simulink model "TST_LogicOperations"  (Simulink 10.0)
settings: Solver=FixedStepDiscrete  StartTime=0.0  StopTime=10.0  FixedStep=0.02  RelTol=1e-3  EnableMultiTasking=on
settings Model: Creator=kharthforeign  LastModifiedBy=unknown
settings DataIOCC: LimitDataPoints=on  SignalLoggingSaveFormat=ModelDataLogs  SaveOutput=off  SignalLogging=off  SaveTime=off
settings OptimizationCC: BlockReduction=off  ConditionallyExecuteInputs=off  OptimizeBlockIOStorage=off  BufferReuse=off  GlobalBufferReuse=off  ExpressionFolding=off  ExpressionDepthLimit=2147483647  LocalBlockOutputs=off  InitFltsAndDblsToZero=on  OptimizeDataStoreBuffers=off  BusAssignmentInplaceUpdate=off
settings DebuggingCC: SolverPrmCheckMsg=warning  FcnCallInpInsideContextMsg=warning  StateNameClashWarn=warning
settings SFSimCC: SimParseCustomCode=off
settings GRTTargetCC: GeneratePreprocessorConditionals=Disable all
settings ConfigComp: CovExternalEMLEnable=off

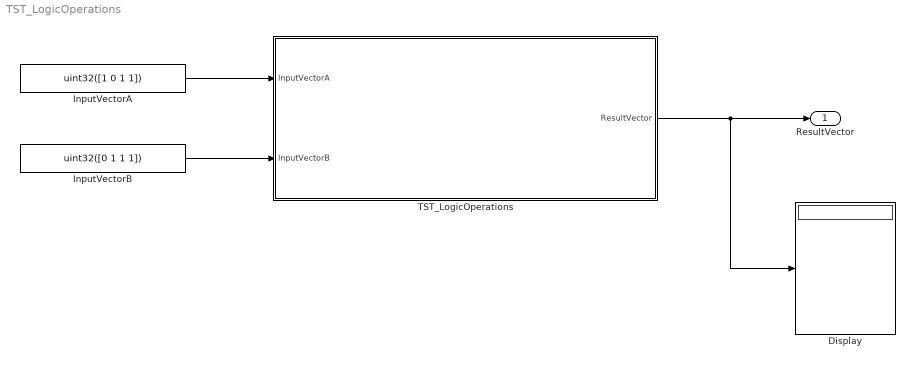
== system TST_LogicOperations ==
  Display : Display
  InputVectorA : Constant  Value=uint32([1 0 1 1])
  InputVectorB : Constant  Value=uint32([0 1 1 1])
  TST_LogicOperations : Subsystem  TreatAsAtomicUnit=on
  ResultVector : Outport
  wires:
  TST_LogicOperations/1(ResultVector) -> ResultVector/1, Display/1
  InputVectorA/1 -> TST_LogicOperations/1(InputVectorA)
  InputVectorB/1 -> TST_LogicOperations/2(InputVectorB)

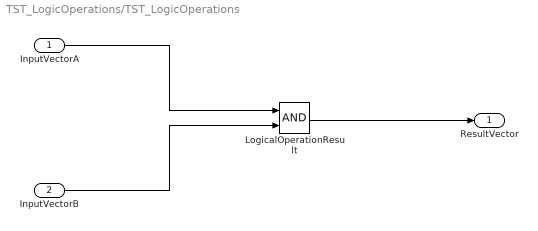
== system TST_LogicOperations/TST_LogicOperations ==
  InputVectorA : Inport
  InputVectorB : Inport  Port=2
  LogicalOperationResult : Logic  AllPortsSameDT=off  OutDataTypeStr=boolean
  ResultVector : Outport
  wires:
  InputVectorA/1 -> LogicalOperationResult/1
  InputVectorB/1 -> LogicalOperationResult/2
  LogicalOperationResult/1 -> ResultVector/1
